simulink model "model2"  (R2021a)
settings: Solver=ode23s  StartTime=0.0  StopTime=0.1  MaxStep=1e-4  RelTol=1e-3
undefined symbols (not defined in the file): D1, Delta, lagging, pulse
libraries: spsVoltageMeasurementLib x23, spsThreePhaseTransformerTwoWindingsLib x22, spsUniversalBridgeLib x18, spsSeriesRLCBranchLib x15, spsRMSLib x13, spsCurrentMeasurementLib x12, spsThreePhaseProgrammableVoltageSourceLib x7, spsGroundLib x5, spsPulseGeneratorThyristor6PulseLib x5, simulink x5, spsThreePhaseTransformerThreeWindingsLib x4, spsControlledCurrentSourceLib x1
settings Model: Creator=Tasneem  LastModifiedBy=Tasneem

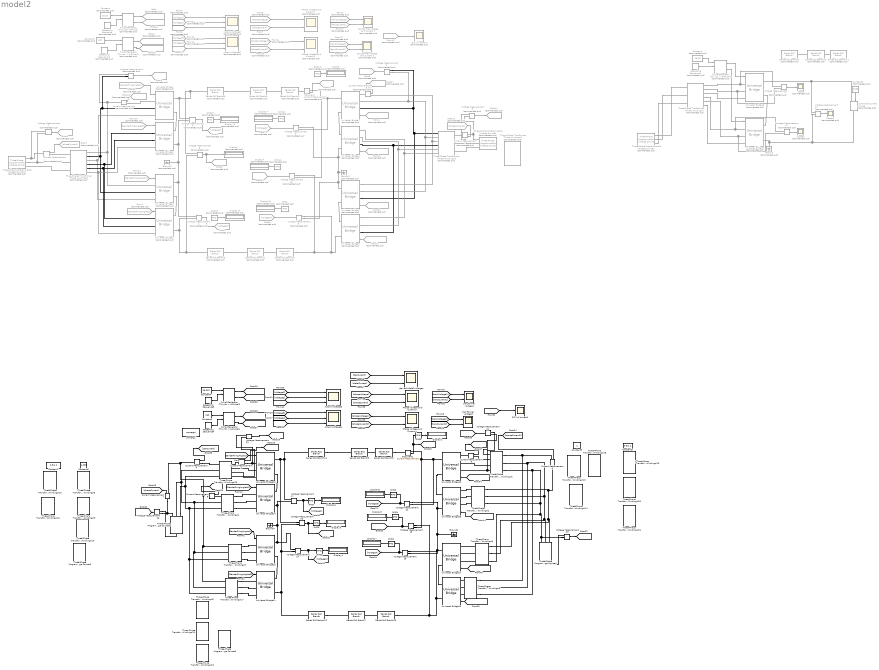
== system model2 ==
  Constant : Constant  Commented=on  Value=18.25
  Constant1 : Constant  Commented=on  Value=18.25
  Constant2 : Constant  Commented=on  Value=160
  Constant3 : Constant  Commented=on  Value=2835
  Constant4 : Constant  Value=28.357
  Constant5 : Constant  Value=160
  Constant6 : Constant  Value=1.025
  Constant7 : Constant  Value=0.9/1.1
  Constant8 : Constant
  Constant9 : Constant  Value=0.9/1.1
  Controlled Current Source : spsControlledCurrentSourceLib/Controlled Current Source  Commented=on  Initialize=on  Source_Type=AC  Amplitude=0  Phase=0  Frequency=0  Measurements=None
  Current Measurement{,1,3,10} (4 alike) : spsCurrentMeasurementLib/Current Measurement  Commented=on  PhasorSimulation=off  OutputType=Complex  PSBequivalent=0
  Current Measurement{2,4..8} (6 alike) : spsCurrentMeasurementLib/Current Measurement  PhasorSimulation=off  OutputType=Complex  PSBequivalent=0
  DC link current : Scope  Commented=on
  DC link current1 : Scope
  DCcurrent : spsCurrentMeasurementLib/Current Measurement  Commented=on  PhasorSimulation=off  OutputType=Complex  PSBequivalent=0
  DCcurrent1 : spsCurrentMeasurementLib/Current Measurement  PhasorSimulation=off  OutputType=Complex  PSBequivalent=0
  Display{,1,5,14..17} (7 alike) : Display  Commented=on
  Display{2..4,6..9} (7 alike) : Display
  From1 : From  Commented=on  GotoTag=SenderFiringAnglesD
  From10 : From  Commented=on  GotoTag=Voltage3
  From11 : From  Commented=on  GotoTag=VoltageSum2
  From12 : From  Commented=on  GotoTag=Voltage4
  From13 : From  Commented=on  GotoTag=transVoltage2
  From14 : From  Commented=on  GotoTag=phaseVoltage2
  From15 : From  Commented=on  GotoTag=phaseCurrent2
  From16 : From  Commented=on  GotoTag=DClinkCurrent
  From17 : From  Commented=on  GotoTag=transCurrent1
  From18 : From  Commented=on  GotoTag=transCurrent2
  From19 : From  Commented=on  GotoTag=ReceiverFiringAnglesD
  From2 : From  Commented=on  GotoTag=ReceiverFiringAnglesY
  From20 : From  Commented=on  GotoTag=ReceiverFiringAnglesY
  From22 : From  Commented=on  GotoTag=SenderFiringAnglesY
  From23 : From  Commented=on  GotoTag=SenderFiringAnglesY
  From24 : From  Commented=on  GotoTag=SenderFiringAnglesD
  From3 : From  Commented=on  GotoTag=ReceiverFiringAnglesD
  From4 : From  Commented=on  GotoTag=Voltage1
  From5 : From  Commented=on  GotoTag=transVoltage1
  From6 : From  Commented=on  GotoTag=phaseVoltage
  From7 : From  Commented=on  GotoTag=phaseCurrent
  From8 : From  Commented=on  GotoTag=VoltageSum1
  From9 : From  Commented=on  GotoTag=Voltage2
  Goto : Goto  Commented=on  GotoTag=SenderFiringAnglesY
  Goto1 : Goto  Commented=on  GotoTag=Voltage2
  Goto10 : Goto  Commented=on  GotoTag=Voltage3
  Goto11 : Goto  Commented=on  GotoTag=phaseVoltage2
  Goto12 : Goto  Commented=on  GotoTag=VoltageSum2
  Goto13 : Goto  Commented=on  GotoTag=phaseCurrent2
  Goto14 : Goto  Commented=on  GotoTag=DClinkCurrent
  Goto15 : Goto  Commented=on  GotoTag=transCurrent1
  Goto16 : Goto  Commented=on  GotoTag=SenderFiringAnglesD
  Goto17 : Goto  Commented=on  GotoTag=transCurrent2
  Goto18 : Goto  Commented=on  GotoTag=ReceiverFiringAnglesD
  Goto2 : Goto  Commented=on  GotoTag=ReceiverFiringAnglesY
  Goto3 : Goto  Commented=on  GotoTag=transVoltage1
  Goto4 : Goto  Commented=on  GotoTag=Voltage1
  Goto5 : Goto  Commented=on  GotoTag=phaseVoltage
  Goto6 : Goto  Commented=on  GotoTag=VoltageSum1
  Goto7 : Goto  Commented=on  GotoTag=phaseCurrent
  Goto8 : Goto  Commented=on  GotoTag=Voltage4
  Goto9 : Goto  Commented=on  GotoTag=transVoltage2
  Ground : spsGroundLib/Ground  Commented=on  LConnTagsString=a
  Ground1 : spsGroundLib/Ground  Commented=on  LConnTagsString=a
  Ground2 : spsGroundLib/Ground  LConnTagsString=a
  Ground3 : spsGroundLib/Ground  Commented=on  LConnTagsString=a
  Ground4 : spsGroundLib/Ground  LConnTagsString=a
  Phase Voltage and Current 1 : Scope  Commented=on  NumInputPorts=2
  Phase Voltage and Current 2 : Scope  Commented=on  NumInputPorts=2
  Phase Voltage and Current 3 : Scope  NumInputPorts=2
  Phase Voltage and Current 4 : Scope  NumInputPorts=2
  "Pulse Generator (Thyristor, 6-Pulse)" : spsPulseGeneratorThyristor6PulseLib/Pulse Generator (Thyristor, 6-Pulse)  Commented=on  GenType=12-pulse  Delta=D1 (lagging)  pwidth=60  Double_Pulse=on  Ts=0
      settings: SourceProductBaseCode=PS
  "Pulse Generator (Thyristor, 6-Pulse)1" : spsPulseGeneratorThyristor6PulseLib/Pulse Generator (Thyristor, 6-Pulse)  Commented=on  GenType=12-pulse  Delta=D1 (lagging)  pwidth=60  Double_Pulse=on  Ts=0
      settings: SourceProductBaseCode=PS
  "Pulse Generator (Thyristor, 6-Pulse)2" : spsPulseGeneratorThyristor6PulseLib/Pulse Generator (Thyristor, 6-Pulse)  Commented=on  GenType=12-pulse  Delta=D1 (lagging)  pwidth=60  Double_Pulse=on  Ts=0
      settings: SourceProductBaseCode=PS
  "Pulse Generator (Thyristor, 6-Pulse)3" : spsPulseGeneratorThyristor6PulseLib/Pulse Generator (Thyristor, 6-Pulse)  GenType=12-pulse  Delta=D1 (lagging)  pwidth=60  Double_Pulse=on  Ts=0
      settings: SourceProductBaseCode=PS
  "Pulse Generator (Thyristor, 6-Pulse)4" : spsPulseGeneratorThyristor6PulseLib/Pulse Generator (Thyristor, 6-Pulse)  GenType=12-pulse  Delta=D1 (lagging)  pwidth=60  Double_Pulse=on  Ts=0
      settings: SourceProductBaseCode=PS
  RMS1 : spsRMSLib/RMS  Commented=on  TrueRMS=on  Freq=60  RMSInit=120  Ts=0
  RMS10 : spsRMSLib/RMS  Commented=on  TrueRMS=on  Freq=50  RMSInit=120  Ts=0
  RMS11 : spsRMSLib/RMS  Commented=on  TrueRMS=on  Freq=60  RMSInit=120  Ts=0
  RMS12 : spsRMSLib/RMS  Commented=on  TrueRMS=on  Freq=60  RMSInit=120  Ts=0
  RMS13 : spsRMSLib/RMS  Commented=on  TrueRMS=on  Freq=50  RMSInit=120  Ts=0
  RMS15 : spsRMSLib/RMS  Commented=on  TrueRMS=on  Freq=50  RMSInit=120  Ts=0
  RMS2 : spsRMSLib/RMS  TrueRMS=on  Freq=60  RMSInit=120  Ts=0
  RMS{3,6..7,9} (4 alike) : spsRMSLib/RMS  TrueRMS=on  Freq=50  RMSInit=120  Ts=0
  RMS4 : spsRMSLib/RMS  TrueRMS=on  Freq=60  RMSInit=120  Ts=0
  RMS5 : spsRMSLib/RMS  TrueRMS=on  Freq=60  RMSInit=120  Ts=0
  Repeating Sequence : simulink/Sources/Repeating Sequence  Commented=on  rep_seq_t=[0 1/50]  rep_seq_y=[0 2*pi]
  Repeating Sequence1 : simulink/Sources/Repeating Sequence  Commented=on  rep_seq_t=[0 1/50]  rep_seq_y=[0 2*pi]
  Repeating Sequence2 : simulink/Sources/Repeating Sequence  Commented=on  rep_seq_t=[0 1/60]  rep_seq_y=[0 2*pi]
  Repeating Sequence3 : simulink/Sources/Repeating Sequence  rep_seq_t=[0 1/50]  rep_seq_y=[0 2*pi]
  Repeating Sequence4 : simulink/Sources/Repeating Sequence  rep_seq_t=[0 1/60]  rep_seq_y=[0 2*pi]
  Scope : Scope  Commented=on
  Scope1 : Scope  Commented=on
  Scope2 : Scope  Commented=on
  Series RLC Branch : spsSeriesRLCBranchLib/Series RLC Branch  Commented=on  LConnTagsString=__new0  RConnTagsString=__new0  BranchType=R  Resistance=10  Inductance=1e-3  SetiL0=off  InitialCurrent=0  Capacitance=1e-6  Setx0=off  InitialVoltage=0  Measurements=None
  Series RLC Branch1 : spsSeriesRLCBranchLib/Series RLC Branch  Commented=on  LConnTagsString=__new0  RConnTagsString=__new0  BranchType=R  Resistance=10  Inductance=1e-3  SetiL0=off  InitialCurrent=0  Capacitance=1e-6  Setx0=off  InitialVoltage=0  Measurements=None
  Series RLC Branch10 : spsSeriesRLCBranchLib/Series RLC Branch  Commented=on  LConnTagsString=__new0  RConnTagsString=__new0  BranchType=R  Resistance=10  Inductance=1e-3  SetiL0=off  InitialCurrent=0  Capacitance=1e-6  Setx0=off  InitialVoltage=0  Measurements=None
  Series RLC Branch11 : spsSeriesRLCBranchLib/Series RLC Branch  Commented=on  LConnTagsString=__new0  RConnTagsString=__new0  BranchType=L  Resistance=1  Inductance=0.1  SetiL0=off  InitialCurrent=0  Capacitance=1e-6  Setx0=off  InitialVoltage=0  Measurements=None
  Series RLC Branch{8,12..14} (4 alike) : spsSeriesRLCBranchLib/Series RLC Branch  LConnTagsString=__new0  RConnTagsString=__new0  BranchType=L  Resistance=10  Inductance=0.1  SetiL0=off  InitialCurrent=0  Capacitance=1e-6  Setx0=off  InitialVoltage=0  Measurements=None
  Series RLC Branch{2,4..6} (4 alike) : spsSeriesRLCBranchLib/Series RLC Branch  Commented=on  LConnTagsString=__new0  RConnTagsString=__new0  BranchType=L  Resistance=10  Inductance=0.1  SetiL0=off  InitialCurrent=0  Capacitance=1e-6  Setx0=off  InitialVoltage=0  Measurements=None
  Series RLC Branch3 : spsSeriesRLCBranchLib/Series RLC Branch  LConnTagsString=__new0  RConnTagsString=__new0  BranchType=R  Resistance=10  Inductance=1e-3  SetiL0=off  InitialCurrent=0  Capacitance=1e-6  Setx0=off  InitialVoltage=0  Measurements=None
  Series RLC Branch7 : spsSeriesRLCBranchLib/Series RLC Branch  LConnTagsString=__new0  RConnTagsString=__new0  BranchType=R  Resistance=10  Inductance=1e-3  SetiL0=off  InitialCurrent=0  Capacitance=1e-6  Setx0=off  InitialVoltage=0  Measurements=None
  Series RLC Branch9 : spsSeriesRLCBranchLib/Series RLC Branch  Commented=on  LConnTagsString=__new0  RConnTagsString=__new0  BranchType=L  Resistance=1  Inductance=0.1  SetiL0=off  InitialCurrent=0  Capacitance=1e-6  Setx0=off  InitialVoltage=0  Measurements=None
  Three-Phase Programmable Voltage Source1 : spsThreePhaseProgrammableVoltageSourceLib/Three-Phase Programmable Voltage Source  Commented=on  PositiveSequence="[22e3*1.025  0 50]"  VariationEntity=None  VariationType=Table of time-amplitude pairs  VariationTypeAlt=Step  VariationStep=0.5  VariationRate=10  VariationMagnitude=0.3  VariationFrequency=2  VariationTiming=[1 2]  VariationPhaseA=off  Amplitudes=[1 0.8 1.2 1.0]  TimeValues=[0 0.1 0.15 0.2]  HarmonicGeneration=off  HarmonicA=[3 0.2 -25 0]  HarmonicB=[2 0.15 35 2]  Timing="[0.05  3]"  BusType=swing  Pref=0  Qref=0  Qmin=-inf  Qmax=inf
  Three-Phase Programmable Voltage Source10 : spsThreePhaseProgrammableVoltageSourceLib/Three-Phase Programmable Voltage Source  Commented=on  PositiveSequence="[22e3*1.025  0 50]"  VariationEntity=None  VariationType=Table of time-amplitude pairs  VariationTypeAlt=Step  VariationStep=0.5  VariationRate=10  VariationMagnitude=0.3  VariationFrequency=2  VariationTiming=[1 2]  VariationPhaseA=off  Amplitudes=[1 0.8 1.2 1.0]  TimeValues=[0 0.1 0.15 0.2]  HarmonicGeneration=off  HarmonicA=[3 0.2 -25 0]  HarmonicB=[2 0.15 35 2]  Timing="[0.05  3]"  BusType=swing  Pref=0  Qref=0  Qmin=-inf  Qmax=inf
  Three-Phase Programmable Voltage Source2 : spsThreePhaseProgrammableVoltageSourceLib/Three-Phase Programmable Voltage Source  PositiveSequence="[22e3  0 50]"  VariationEntity=None  VariationType=Table of time-amplitude pairs  VariationTypeAlt=Step  VariationStep=0.5  VariationRate=10  VariationMagnitude=0.3  VariationFrequency=2  VariationTiming=[1 2]  VariationPhaseA=off  Amplitudes=[1 0.8 1.2 1.0]  TimeValues=[0 0.1 0.15 0.2]  HarmonicGeneration=off  HarmonicA=[3 0.2 -25 0]  HarmonicB=[2 0.15 35 2]  Timing="[0.05  3]"  BusType=swing  Pref=0  Qref=0  Qmin=-inf  Qmax=inf
  Three-Phase Programmable Voltage Source3 : spsThreePhaseProgrammableVoltageSourceLib/Three-Phase Programmable Voltage Source  Commented=on  PositiveSequence="[20e3  0 60]"  VariationEntity=None  VariationType=Table of time-amplitude pairs  VariationTypeAlt=Step  VariationStep=0.5  VariationRate=10  VariationMagnitude=0.3  VariationFrequency=2  VariationTiming=[1 2]  VariationPhaseA=off  Amplitudes=[1 0.8 1.2 1.0]  TimeValues=[0 0.1 0.15 0.2]  HarmonicGeneration=off  HarmonicA=[3 0.2 -25 0]  HarmonicB=[2 0.15 35 2]  Timing="[0.05  3]"  BusType=swing  Pref=0  Qref=0  Qmin=-inf  Qmax=inf
  Three-Phase Programmable Voltage Source4 : spsThreePhaseProgrammableVoltageSourceLib/Three-Phase Programmable Voltage Source  PositiveSequence="[20e3  0 60]"  VariationEntity=None  VariationType=Table of time-amplitude pairs  VariationTypeAlt=Step  VariationStep=0.5  VariationRate=10  VariationMagnitude=0.3  VariationFrequency=2  VariationTiming=[1 2]  VariationPhaseA=off  Amplitudes=[1 0.8 1.2 1.0]  TimeValues=[0 0.1 0.15 0.2]  HarmonicGeneration=off  HarmonicA=[3 0.2 -25 0]  HarmonicB=[2 0.15 35 2]  Timing="[0.05  3]"  BusType=swing  Pref=0  Qref=0  Qmin=-inf  Qmax=inf
  Three-Phase Programmable Voltage Source5 : spsThreePhaseProgrammableVoltageSourceLib/Three-Phase Programmable Voltage Source  PositiveSequence="[22e3*1.025  0 50]"  VariationEntity=None  VariationType=Table of time-amplitude pairs  VariationTypeAlt=Step  VariationStep=0.5  VariationRate=10  VariationMagnitude=0.3  VariationFrequency=2  VariationTiming=[1 2]  VariationPhaseA=off  Amplitudes=[1 0.8 1.2 1.0]  TimeValues=[0 0.1 0.15 0.2]  HarmonicGeneration=off  HarmonicA=[3 0.2 -25 0]  HarmonicB=[2 0.15 35 2]  Timing="[0.05  3]"  BusType=swing  Pref=0  Qref=0  Qmin=-inf  Qmax=inf
  Three-Phase Programmable Voltage Source6 : spsThreePhaseProgrammableVoltageSourceLib/Three-Phase Programmable Voltage Source  PositiveSequence="[22e3  0 50]"  VariationEntity=None  VariationType=Table of time-amplitude pairs  VariationTypeAlt=Step  VariationStep=0.5  VariationRate=10  VariationMagnitude=0.3  VariationFrequency=2  VariationTiming=[1 2]  VariationPhaseA=off  Amplitudes=[1 0.8 1.2 1.0]  TimeValues=[0 0.1 0.15 0.2]  HarmonicGeneration=off  HarmonicA=[3 0.2 -25 0]  HarmonicB=[2 0.15 35 2]  Timing="[0.05  3]"  BusType=swing  Pref=0  Qref=0  Qmin=-inf  Qmax=inf
  Three-Phase Transformer (Three Windings)1 : spsThreePhaseTransformerThreeWindingsLib/Three-Phase Transformer (Three Windings)  Commented=on  Winding1Connection=Y  Winding2Connection=Y  Winding3Connection=Delta (D1)  CoreType=Three single-phase transformers  SetSaturation=off  Hysteresis=off  DataFile='hysteresis'  SetInitialFlux=off  Measurements=None  UNITS=SI  NominalPower=[ 1600e6 , 50 ]  Winding1=[22e3 0 0]  Winding2=[220e3 0 0]  Winding3=[220e3*sqrt(3) 0.001 0]  Rm=inf  Lm=inf  L0=0.5  Saturation=[0 0;4.2658 1910.3;1777.4 2419.7]  InitialFluxes=[0 87.9108143390969 87.9108143390969]  BreakLoop=off  DiscreteSolver=Trapezoidal iterative  DataType=on  TransfoNumber=1
      settings: SourceProductBaseCode=PS
  Three-Phase Transformer (Three Windings)2 : spsThreePhaseTransformerThreeWindingsLib/Three-Phase Transformer (Three Windings)  Commented=on  Winding1Connection=Y  Winding2Connection=Y  Winding3Connection=Delta (D1)  CoreType=Three single-phase transformers  SetSaturation=off  Hysteresis=off  DataFile='hysteresis'  SetInitialFlux=off  Measurements=None  UNITS=SI  NominalPower=[ 1600e6 , 50 ]  Winding1=[22e3 0 0]  Winding2=[220e3 0 0]  Winding3=[220e3*sqrt(3) 0.001 0]  Rm=inf  Lm=inf  L0=0.5  Saturation=[0 0;4.2658 1910.3;1777.4 2419.7]  InitialFluxes=[0 87.9108143390969 87.9108143390969]  BreakLoop=off  DiscreteSolver=Trapezoidal iterative  DataType=on  TransfoNumber=1
      settings: SourceProductBaseCode=PS
  Three-Phase Transformer (Three Windings)3 : spsThreePhaseTransformerThreeWindingsLib/Three-Phase Transformer (Three Windings)  Commented=on  Winding1Connection=Y  Winding2Connection=Y  Winding3Connection=Delta (D1)  CoreType=Three single-phase transformers  SetSaturation=off  Hysteresis=off  DataFile='hysteresis'  SetInitialFlux=off  Measurements=None  UNITS=SI  NominalPower=[ 18000e6 , 60 ]  Winding1=[20e3 0 0]  Winding2=[200e3 0 0]  Winding3=[200e3*sqrt(3) 0.0001 0]  Rm=inf  Lm=inf  L0=0.5  Saturation=[0 0;0.66653 1910.3;277.72 2419.7]  InitialFluxes=[-43.3164889574264 21.6582444787132 21.6582444787132]  BreakLoop=off  DiscreteSolver=Trapezoidal iterative  DataType=on  TransfoNumber=1
      settings: SourceProductBaseCode=PS
  Three-Phase Transformer (Three Windings)4 : spsThreePhaseTransformerThreeWindingsLib/Three-Phase Transformer (Three Windings)  Commented=on  Winding1Connection=Y  Winding2Connection=Y  Winding3Connection=Delta (D1)  CoreType=Three single-phase transformers  SetSaturation=off  Hysteresis=off  DataFile='hysteresis'  SetInitialFlux=off  Measurements=None  UNITS=SI  NominalPower=[ 1600e6 , 60 ]  Winding1=[20e3 0 0]  Winding2=[200e3 0 0]  Winding3=[200e3*sqrt(3) 0.001 0]  Rm=inf  Lm=inf  L0=0.5  Saturation=[0 0;4.2658 1910.3;1777.4 2419.7]  InitialFluxes=[0 64.9747334361397 64.9747334361397]  BreakLoop=off  DiscreteSolver=Trapezoidal iterative  DataType=on  TransfoNumber=1
      settings: SourceProductBaseCode=PS
  Three-Phase Transformer (Two Windings)1 : spsThreePhaseTransformerTwoWindingsLib/Three-Phase Transformer (Two Windings)  Winding1Connection=Yn  Winding2Connection=Y  CoreType=Three single-phase transformers  SetSaturation=off  Hysteresis=off  DataFile='hysteresis'  SetInitialFlux=off  Measurements=None  UNITS=SI  NominalPower=[ 800e6 , 60 ]  Winding1=[200e3 0.001 0]  Winding2=[20e3 0.001 0]  Rm=inf  Lm=inf  L0=0.5  Saturation=[0 0;17.636 519.8;7348.5 658.41]  InitialFluxes=[0 714.722067624574 714.722315656474]  BreakLoop=off  DiscreteSolver=Trapezoidal iterative  DataType=on  TransfoNumber=1
  Three-Phase Transformer (Two Windings)10 : spsThreePhaseTransformerTwoWindingsLib/Three-Phase Transformer (Two Windings)  Winding1Connection=Y  Winding2Connection=Y  CoreType=Three single-phase transformers  SetSaturation=off  Hysteresis=off  DataFile='hysteresis'  SetInitialFlux=off  Measurements=None  UNITS=SI  NominalPower=[ 800e6 , 50 ]  Winding1=[22e3*1.025 1e-6 0]  Winding2=[220e3*1.025 1e-6 0]  Rm=inf  Lm=inf  L0=0.00044961  Saturation=[0 0;156.42 70.329;65175 89.083]  InitialFluxes=[0 85.766648119398 85.766648119398]  BreakLoop=off  DiscreteSolver=Trapezoidal iterative  DataType=on  TransfoNumber=1
  Three-Phase Transformer (Two Windings)11 : spsThreePhaseTransformerTwoWindingsLib/Three-Phase Transformer (Two Windings)  Winding1Connection=Y  Winding2Connection=Delta (D1)  CoreType=Three single-phase transformers  SetSaturation=off  Hysteresis=off  DataFile='hysteresis'  SetInitialFlux=off  Measurements=None  UNITS=SI  NominalPower=[ 800e6 , 50 ]  Winding1=[22e3 1e-6 0]  Winding2=[220e3 1e-6 0]  Rm=inf  Lm=inf  L0=0.00044961  Saturation=[0 0;156.42 70.329;65175 89.083]  InitialFluxes=[0 85.766648119398 85.766648119398]  BreakLoop=off  DiscreteSolver=Trapezoidal iterative  DataType=on  TransfoNumber=1
  Three-Phase Transformer (Two Windings)12 : spsThreePhaseTransformerTwoWindingsLib/Three-Phase Transformer (Two Windings)  Winding1Connection=Y  Winding2Connection=Y  CoreType=Three single-phase transformers  SetSaturation=off  Hysteresis=off  DataFile='hysteresis'  SetInitialFlux=off  Measurements=None  UNITS=SI  NominalPower=[ 800e6 , 50 ]  Winding1=[22e3 1e-6 0]  Winding2=[220e3 1e-6 0]  Rm=inf  Lm=inf  L0=0.00044961  Saturation=[0 0;156.42 70.329;65175 89.083]  InitialFluxes=[0 85.766648119398 85.766648119398]  BreakLoop=off  DiscreteSolver=Trapezoidal iterative  DataType=on  TransfoNumber=1
  Three-Phase Transformer (Two Windings)13 : spsThreePhaseTransformerTwoWindingsLib/Three-Phase Transformer (Two Windings)  Winding1Connection=Y  Winding2Connection=Y  CoreType=Three single-phase transformers  SetSaturation=off  Hysteresis=off  DataFile='hysteresis'  SetInitialFlux=off  Measurements=None  UNITS=SI  NominalPower=[ 800e6 , 60 ]  Winding1=[200e3 1e-6 0]  Winding2=[20e3 1e-6 0]  Rm=inf  Lm=inf  L0=0.5  Saturation=[0 0;17.636 519.8;7348.5 658.41]  InitialFluxes=[0 714.722067624574 714.722315656474]  BreakLoop=off  DiscreteSolver=Trapezoidal iterative  DataType=on  TransfoNumber=1
  Three-Phase Transformer (Two Windings)14 : spsThreePhaseTransformerTwoWindingsLib/Three-Phase Transformer (Two Windings)  Winding1Connection=Delta (D1)  Winding2Connection=Y  CoreType=Three single-phase transformers  SetSaturation=off  Hysteresis=off  DataFile='hysteresis'  SetInitialFlux=off  Measurements=None  UNITS=SI  NominalPower=[ 800e6 , 60 ]  Winding1=[200e3 1e-6 0]  Winding2=[20e3 1e-6 0]  Rm=inf  Lm=inf  L0=0.5  Saturation=[0 0;17.636 519.8;7348.5 658.41]  InitialFluxes=[0 714.722067624574 714.722315656474]  BreakLoop=off  DiscreteSolver=Trapezoidal iterative  DataType=on  TransfoNumber=1
  Three-Phase Transformer (Two Windings)15 : spsThreePhaseTransformerTwoWindingsLib/Three-Phase Transformer (Two Windings)  Winding1Connection=Y  Winding2Connection=Yn  CoreType=Three single-phase transformers  SetSaturation=off  Hysteresis=off  DataFile='hysteresis'  SetInitialFlux=off  Measurements=None  UNITS=SI  NominalPower=[ 800e6 , 50 ]  Winding1=[22e3 1e-6 0]  Winding2=[220e3*0.9 1e-6 0]  Rm=inf  Lm=inf  L0=0.00044961  Saturation=[0 0;156.42 70.329;65175 89.083]  InitialFluxes=[0 85.766648119398 85.766648119398]  BreakLoop=off  DiscreteSolver=Trapezoidal iterative  DataType=on  TransfoNumber=1
  Three-Phase Transformer (Two Windings)16 : spsThreePhaseTransformerTwoWindingsLib/Three-Phase Transformer (Two Windings)  Winding1Connection=Y  Winding2Connection=Delta (D1)  CoreType=Three single-phase transformers  SetSaturation=off  Hysteresis=off  DataFile='hysteresis'  SetInitialFlux=off  Measurements=None  UNITS=SI  NominalPower=[ 800e6 , 50 ]  Winding1=[22e3 1e-6 0]  Winding2=[220e3*0.9 1e-6 0]  Rm=inf  Lm=inf  L0=0.00044961  Saturation=[0 0;156.42 70.329;65175 89.083]  InitialFluxes=[0 85.766648119398 85.766648119398]  BreakLoop=off  DiscreteSolver=Trapezoidal iterative  DataType=on  TransfoNumber=1
  Three-Phase Transformer (Two Windings)17 : spsThreePhaseTransformerTwoWindingsLib/Three-Phase Transformer (Two Windings)  Winding1Connection=Y  Winding2Connection=Delta (D1)  CoreType=Three single-phase transformers  SetSaturation=off  Hysteresis=off  DataFile='hysteresis'  SetInitialFlux=off  Measurements=None  UNITS=SI  NominalPower=[ 800e6 , 50 ]  Winding1=[22e3 1e-6 0]  Winding2=[220e3 1e-6 0]  Rm=inf  Lm=inf  L0=0.00044961  Saturation=[0 0;156.42 70.329;65175 89.083]  InitialFluxes=[0 85.766648119398 85.766648119398]  BreakLoop=off  DiscreteSolver=Trapezoidal iterative  DataType=on  TransfoNumber=1
  Three-Phase Transformer (Two Windings)18 : spsThreePhaseTransformerTwoWindingsLib/Three-Phase Transformer (Two Windings)  Winding1Connection=Yn  Winding2Connection=Y  CoreType=Three single-phase transformers  SetSaturation=off  Hysteresis=off  DataFile='hysteresis'  SetInitialFlux=off  Measurements=None  UNITS=SI  NominalPower=[ 800e6 , 60 ]  Winding1=[200e3 1e-6 0]  Winding2=[20e3 1e-6 0]  Rm=inf  Lm=inf  L0=0.5  Saturation=[0 0;17.636 519.8;7348.5 658.41]  InitialFluxes=[0 714.722067624574 714.722315656474]  BreakLoop=off  DiscreteSolver=Trapezoidal iterative  DataType=on  TransfoNumber=1
  Three-Phase Transformer (Two Windings)19 : spsThreePhaseTransformerTwoWindingsLib/Three-Phase Transformer (Two Windings)  Winding1Connection=Yn  Winding2Connection=Y  CoreType=Three single-phase transformers  SetSaturation=off  Hysteresis=off  DataFile='hysteresis'  SetInitialFlux=off  Measurements=None  UNITS=SI  NominalPower=[ 800e6 , 60 ]  Winding1=[200e3*1.1 1e-6 0]  Winding2=[20e3 1e-6 0]  Rm=inf  Lm=inf  L0=0.5  Saturation=[0 0;17.636 519.8;7348.5 658.41]  InitialFluxes=[0 714.722067624574 714.722315656474]  BreakLoop=off  DiscreteSolver=Trapezoidal iterative  DataType=on  TransfoNumber=1
  Three-Phase Transformer (Two Windings)2 : spsThreePhaseTransformerTwoWindingsLib/Three-Phase Transformer (Two Windings)  Winding1Connection=Delta (D1)  Winding2Connection=Y  CoreType=Three single-phase transformers  SetSaturation=off  Hysteresis=off  DataFile='hysteresis'  SetInitialFlux=off  Measurements=None  UNITS=SI  NominalPower=[ 800e6 , 60 ]  Winding1=[200e3 1e-6 0]  Winding2=[20e3 1e-6 0]  Rm=inf  Lm=inf  L0=0.5  Saturation=[0 0;17.636 519.8;7348.5 658.41]  InitialFluxes=[0 714.722067624574 714.722315656474]  BreakLoop=off  DiscreteSolver=Trapezoidal iterative  DataType=on  TransfoNumber=1
  Three-Phase Transformer (Two Windings)20 : spsThreePhaseTransformerTwoWindingsLib/Three-Phase Transformer (Two Windings)  Winding1Connection=Delta (D1)  Winding2Connection=Y  CoreType=Three single-phase transformers  SetSaturation=off  Hysteresis=off  DataFile='hysteresis'  SetInitialFlux=off  Measurements=None  UNITS=SI  NominalPower=[ 800e6 , 60 ]  Winding1=[200e3*1.1 1e-6 0]  Winding2=[20e3 1e-6 0]  Rm=inf  Lm=inf  L0=0.5  Saturation=[0 0;17.636 519.8;7348.5 658.41]  InitialFluxes=[0 714.722067624574 714.722315656474]  BreakLoop=off  DiscreteSolver=Trapezoidal iterative  DataType=on  TransfoNumber=1
  Three-Phase Transformer (Two Windings)21 : spsThreePhaseTransformerTwoWindingsLib/Three-Phase Transformer (Two Windings)  Winding1Connection=Y  Winding2Connection=Y  CoreType=Three single-phase transformers  SetSaturation=off  Hysteresis=off  DataFile='hysteresis'  SetInitialFlux=off  Measurements=None  UNITS=SI  NominalPower=[ 800e6 , 60 ]  Winding1=[200e3*1.1 0.0001 0]  Winding2=[20e3 0.0001 0]  Rm=inf  Lm=inf  L0=0.5  Saturation=[0 0;17.636 519.8;7348.5 658.41]  InitialFluxes=[0 714.722067624574 714.722315656474]  BreakLoop=off  DiscreteSolver=Trapezoidal iterative  DataType=on  TransfoNumber=1
  Three-Phase Transformer (Two Windings)23 : spsThreePhaseTransformerTwoWindingsLib/Three-Phase Transformer (Two Windings)  Winding1Connection=Y  Winding2Connection=Yn  CoreType=Three single-phase transformers  SetSaturation=off  Hysteresis=off  DataFile='hysteresis'  SetInitialFlux=off  Measurements=None  UNITS=SI  NominalPower=[ 800e6 , 50 ]  Winding1=[22e3 1e-6 0]  Winding2=[220e3 1e-6 0]  Rm=inf  Lm=inf  L0=0.00044961  Saturation=[0 0;156.42 70.329;65175 89.083]  InitialFluxes=[0 85.766648119398 85.766648119398]  BreakLoop=off  DiscreteSolver=Trapezoidal iterative  DataType=on  TransfoNumber=1
  Three-Phase Transformer (Two Windings)3 : spsThreePhaseTransformerTwoWindingsLib/Three-Phase Transformer (Two Windings)  Winding1Connection=Y  Winding2Connection=Yn  CoreType=Three single-phase transformers  SetSaturation=off  Hysteresis=off  DataFile='hysteresis'  SetInitialFlux=off  Measurements=None  UNITS=SI  NominalPower=[ 800e6 , 50 ]  Winding1=[22e3 1e-6 0]  Winding2=[220e3 1e-6 0]  Rm=inf  Lm=inf  L0=0.00044961  Saturation=[0 0;156.42 70.329;65175 89.083]  InitialFluxes=[0 85.766648119398 85.766648119398]  BreakLoop=off  DiscreteSolver=Trapezoidal iterative  DataType=on  TransfoNumber=1
  Three-Phase Transformer (Two Windings)4 : spsThreePhaseTransformerTwoWindingsLib/Three-Phase Transformer (Two Windings)  Winding1Connection=Y  Winding2Connection=Delta (D1)  CoreType=Three single-phase transformers  SetSaturation=off  Hysteresis=off  DataFile='hysteresis'  SetInitialFlux=off  Measurements=None  UNITS=SI  NominalPower=[ 800e6 , 50 ]  Winding1=[22e3 1e-6 0]  Winding2=[220e3 1e-6 0]  Rm=inf  Lm=inf  L0=0.00044961  Saturation=[0 0;156.42 70.329;65175 89.083]  InitialFluxes=[0 85.766648119398 85.766648119398]  BreakLoop=off  DiscreteSolver=Trapezoidal iterative  DataType=on  TransfoNumber=1
  Three-Phase Transformer (Two Windings)5 : spsThreePhaseTransformerTwoWindingsLib/Three-Phase Transformer (Two Windings)  Winding1Connection=Y  Winding2Connection=Yn  CoreType=Three single-phase transformers  SetSaturation=off  Hysteresis=off  DataFile='hysteresis'  SetInitialFlux=off  Measurements=None  UNITS=SI  NominalPower=[ 800e6 , 50 ]  Winding1=[22e3*1.025 1e-6 0]  Winding2=[220e3*1.025 1e-6 0]  Rm=inf  Lm=inf  L0=0.00044961  Saturation=[0 0;156.42 70.329;65175 89.083]  InitialFluxes=[0 85.766648119398 85.766648119398]  BreakLoop=off  DiscreteSolver=Trapezoidal iterative  DataType=on  TransfoNumber=1
  Three-Phase Transformer (Two Windings)6 : spsThreePhaseTransformerTwoWindingsLib/Three-Phase Transformer (Two Windings)  Winding1Connection=Y  Winding2Connection=Y  CoreType=Three single-phase transformers  SetSaturation=off  Hysteresis=off  DataFile='hysteresis'  SetInitialFlux=off  Measurements=None  UNITS=SI  NominalPower=[ 800e6 , 60 ]  Winding1=[200e3 0.001 0]  Winding2=[20e3 0.001 0]  Rm=inf  Lm=inf  L0=0.5  Saturation=[0 0;17.636 519.8;7348.5 658.41]  InitialFluxes=[0 714.722067624574 714.722315656474]  BreakLoop=off  DiscreteSolver=Trapezoidal iterative  DataType=on  TransfoNumber=1
  Three-Phase Transformer (Two Windings)7 : spsThreePhaseTransformerTwoWindingsLib/Three-Phase Transformer (Two Windings)  Winding1Connection=Y  Winding2Connection=Y  CoreType=Three single-phase transformers  SetSaturation=off  Hysteresis=off  DataFile='hysteresis'  SetInitialFlux=off  Measurements=None  UNITS=SI  NominalPower=[ 800e6 , 50 ]  Winding1=[22e3 1e-6 0]  Winding2=[220e3 1e-6 0]  Rm=inf  Lm=inf  L0=0.00044961  Saturation=[0 0;156.42 70.329;65175 89.083]  InitialFluxes=[0 85.766648119398 85.766648119398]  BreakLoop=off  DiscreteSolver=Trapezoidal iterative  DataType=on  TransfoNumber=1
  Three-Phase Transformer (Two Windings)8 : spsThreePhaseTransformerTwoWindingsLib/Three-Phase Transformer (Two Windings)  Winding1Connection=Delta (D1)  Winding2Connection=Y  CoreType=Three single-phase transformers  SetSaturation=off  Hysteresis=off  DataFile='hysteresis'  SetInitialFlux=off  Measurements=None  UNITS=SI  NominalPower=[ 800e6 , 60 ]  Winding1=[200e3 1e-6 0]  Winding2=[20e3 1e-6 0]  Rm=inf  Lm=inf  L0=0.5  Saturation=[0 0;17.636 519.8;7348.5 658.41]  InitialFluxes=[0 714.722067624574 714.722315656474]  BreakLoop=off  DiscreteSolver=Trapezoidal iterative  DataType=on  TransfoNumber=1
  Three-Phase Transformer (Two Windings)9 : spsThreePhaseTransformerTwoWindingsLib/Three-Phase Transformer (Two Windings)  Winding1Connection=Y  Winding2Connection=Delta (D1)  CoreType=Three single-phase transformers  SetSaturation=off  Hysteresis=off  DataFile='hysteresis'  SetInitialFlux=off  Measurements=None  UNITS=SI  NominalPower=[ 800e6 , 50 ]  Winding1=[22e3*1.025 1e-6 0]  Winding2=[220e3*1.025 1e-6 0]  Rm=inf  Lm=inf  L0=0.00044961  Saturation=[0 0;156.42 70.329;65175 89.083]  InitialFluxes=[0 85.766648119398 85.766648119398]  BreakLoop=off  DiscreteSolver=Trapezoidal iterative  DataType=on  TransfoNumber=1
  Universal Bridge{,1..9} (10 alike) : spsUniversalBridgeLib/Universal Bridge  Commented=on  Arms=3  SnubberResistance=1e5  SnubberCapacitance=inf  Device=Thyristors  Ron=1e-9  Lon=0  ForwardVoltages="[  0  0  ]"  ForwardVoltage=0  GTOparameters=[ 10e-6 , 20e-6 ]  IGBTparameters=[ 1e-6 , 2e-6 ]  Measurements=None  Measurements_2=None  converterType=Rectifier
  Universal Bridge{10..17} (8 alike) : spsUniversalBridgeLib/Universal Bridge  Arms=3  SnubberResistance=1e5  SnubberCapacitance=inf  Device=Thyristors  Ron=1e-9  Lon=0  ForwardVoltages="[  0  0  ]"  ForwardVoltage=0  GTOparameters=[ 10e-6 , 20e-6 ]  IGBTparameters=[ 1e-6 , 2e-6 ]  Measurements=None  Measurements_2=None  converterType=Rectifier
  Voltage Measurement{,1..12} (13 alike) : spsVoltageMeasurementLib/Voltage Measurement  Commented=on  PhasorSimulation=off  OutputType=Complex  PSBequivalent=0
  Voltage Measurement{13..22} (10 alike) : spsVoltageMeasurementLib/Voltage Measurement  PhasorSimulation=off  OutputType=Complex  PSBequivalent=0
  output voltages1 : Scope  Commented=on  NumInputPorts=3
  output voltages2 : Scope  Commented=on  NumInputPorts=3
  output voltages3 : Scope  NumInputPorts=3
  output voltages4 : Scope  NumInputPorts=3
  powergui : spspowerguiLib/powergui  Priority=1  SimulationMode=Discrete  SampleTime=1e-6  frequency=60  Iterations=50  frequencyindice=0  Pbase=100e6  ErrMax=1e-4  UnitsV=kV  UnitsW=MW  buscounter=0  FunctionMessages=off  echomessages=off  EnableUseOfTLC=off  CurrentSourceSwitches=off  DisableSnubberDevices=off  DisableRonSwitches=off  DisableVfSwitches=off  DisplayEquations=off  AutomaticDiscreteSolvers=off  SolverType=Tustin/Backward Euler (TBE)  Interpol=off  ExternalGateDelay=off  methode=off  Ts=100  x0status=blocks  SPID=on  SwTol=0  HookPort=off  NonlinearTolerance=1e-4  nMaxIteration=100  ContinueOnMaxIteration=off  RestoreLinks=warning  ResistiveCurrentMeasurement=off  Frange=[0:2:500]  Ylog=off  Xlog=on  ShowGrid=off  save=off  variable=ZData  structure=0  ZoomFFT=off  StartTime=0.0  cycles=1  DisplayStyle=1  fundamental=60  FreqAxis=off  MaxFrequency=1000  frequencyindicesteady=1  RmsSteady=1  display=off
  star and delta voltages : Scope  NumInputPorts=2
  transformer voltage and current 1 : Scope  Commented=on  NumInputPorts=2
  transformer voltage and current 2 : Scope  Commented=on  NumInputPorts=2
  transformer voltage1 : Scope  NumInputPorts=2
  transformer voltage2 : Scope  NumInputPorts=2
  wires:
  Voltage Measurement2/1 -> Goto5/1
  RMS11/1 -> Display5/1
  RMS15/1 -> Display15/1
  RMS10/1 -> Display14/1
  Current Measurement10/1 -> Goto17/1
  RMS1/1 -> Display16/1
  From3/1 -> Universal Bridge3/1
  DCcurrent/1 -> Goto14/1
  From15/1 -> Phase Voltage and Current 2/2  "phase current 2"
  From13/1 -> transformer voltage and current 2/1  "transVotage2"
  Voltage Measurement6/1 -> Goto8/1
  Voltage Measurement9/1 -> Goto10/1
  Voltage Measurement10/1 -> Goto12/1
  From12/1 -> output voltages2/2  "bottom right voltage"
  From10/1 -> output voltages2/1  "upper right voltage"
  From8/1 -> output voltages1/3  "total left voltage"
  From4/1 -> output voltages1/1  "upper  left voltage"
  From9/1 -> output voltages1/2  "bottom left voltage"
  Constant2/1 -> "Pulse Generator (Thyristor, 6-Pulse)2"/1
  From7/1 -> Phase Voltage and Current 1/2  "phase current 1"
  "Pulse Generator (Thyristor, 6-Pulse)"/1 -> Goto/1
  Repeating Sequence/1 -> "Pulse Generator (Thyristor, 6-Pulse)"/2
  Voltage Measurement4/1 -> Goto4/1
  Voltage Measurement5/1 -> Display1/1, Goto6/1
  Voltage Measurement8/1 -> Goto9/1
  "Pulse Generator (Thyristor, 6-Pulse)2"/1 -> Goto2/1
  From6/1 -> Phase Voltage and Current 1/1  "phase voltage 1"
  From5/1 -> transformer voltage and current 1/1  "transVoltage1"
  Constant/1 -> "Pulse Generator (Thyristor, 6-Pulse)"/1
  From17/1 -> transformer voltage and current 1/2  "transCurrent1"
  From16/1 -> DC link current/1  "DC link current"
  Repeating Sequence2/1 -> "Pulse Generator (Thyristor, 6-Pulse)2"/2
  RMS12/1 -> Display17/1
  From18/1 -> transformer voltage and current 2/2  "transCurrent2"
  From14/1 -> Phase Voltage and Current 2/1  "phase voltage 2"
  Voltage Measurement/1 -> Goto3/1
  From1/1 -> Universal Bridge1/1
  From11/1 -> output voltages2/3  "total right voltage"
  From2/1 -> Universal Bridge2/1
  RMS13/1 -> Display/1
  From19/1 -> Universal Bridge4/1
  From20/1 -> Universal Bridge5/1
  From22/1 -> Universal Bridge7/1
  From24/1 -> Universal Bridge6/1
  From23/1 -> Universal Bridge/1
  Current Measurement1/1 -> Goto7/1
  Current Measurement3/1 -> Goto13/1
  Voltage Measurement3/1 -> Goto11/1
  "Pulse Generator (Thyristor, 6-Pulse)"/2 -> Goto16/1
  "Pulse Generator (Thyristor, 6-Pulse)2"/2 -> Goto18/1
  Current Measurement/1 -> Goto15/1
  Voltage Measurement1/1 -> Goto1/1
  Constant1/1 -> "Pulse Generator (Thyristor, 6-Pulse)1"/1
  Repeating Sequence1/1 -> "Pulse Generator (Thyristor, 6-Pulse)1"/2
  "Pulse Generator (Thyristor, 6-Pulse)1"/1 -> Universal Bridge8/1
  "Pulse Generator (Thyristor, 6-Pulse)1"/2 -> Universal Bridge9/1
  Constant3/1 -> Controlled Current Source/1
  Voltage Measurement7/1 -> Scope/1
  Voltage Measurement12/1 -> Scope2/1
  Voltage Measurement11/1 -> Scope1/1
  Voltage Measurement16/1 -> [phaseVoltage]
  DCcurrent1/1 -> RMS6/1, [DClinkCurrent]
  RMS6/1 -> Display2/1
  RMS2/1 -> Display7/1
  RMS4/1 -> Display9/1
  RMS5/1 -> Display8/1
  RMS3/1 -> Display4/1
  RMS9/1 -> Display3/1
  RMS7/1 -> Display6/1
  [ReceiverFiringAnglesY] -> Universal Bridge12/1
  [ReceiverFiringAnglesD] -> Universal Bridge13/1
  Voltage Measurement18/1 -> [VoltageSum1], RMS9/1
  Current Measurement2/1 -> [transCurrent1]
  [transCurrent2] -> transformer voltage2/2  "transCurrent2"
  [transCurrent1] -> transformer voltage1/2  "transCurrent1"
  Voltage Measurement13/1 -> [transVoltage1]
  [DClinkCurrent] -> DC link current1/1  "DC link current"
  [phaseCurrent2] -> Phase Voltage and Current 4/2  "phase current 2"
  [phaseVoltage2] -> Phase Voltage and Current 4/1  "phase voltage 2"
  Current Measurement6/1 -> [phaseCurrent2]
  Voltage Measurement19/1 -> [Voltage4], RMS2/1
  Voltage Measurement21/1 -> [transVoltage2]
  [transVoltage2] -> transformer voltage2/1  "transVotage2"
  Voltage Measurement22/1 -> [Voltage3], RMS5/1
  Voltage Measurement15/1 -> [VoltageSum2], RMS4/1
  [Voltage3] -> output voltages4/1  "upper right voltage"
  [Voltage4] -> output voltages4/2  "bottom right voltage"
  [VoltageSum2] -> output voltages4/3  "total right voltage"
  [VoltageSum1] -> output voltages3/3  "total left voltage"
  Voltage Measurement17/1 -> [Voltage1], RMS7/1
  [Voltage2] -> output voltages3/2  "bottom left voltage"
  [transVoltage1] -> transformer voltage1/1  "transVoltage1"
  [Voltage1] -> output voltages3/1  "upper  left voltage"
  Voltage Measurement14/1 -> [Voltage2], RMS3/1
  [phaseVoltage] -> Phase Voltage and Current 3/1  "phase voltage 1"
  [phaseCurrent] -> Phase Voltage and Current 3/2  "phase current 1"
  Constant5/1 -> "Pulse Generator (Thyristor, 6-Pulse)4"/1
  Repeating Sequence4/1 -> "Pulse Generator (Thyristor, 6-Pulse)4"/2
  "Pulse Generator (Thyristor, 6-Pulse)4"/1 -> [ReceiverFiringAnglesY]
  [SenderFiringAnglesD] -> Universal Bridge11/1
  "Pulse Generator (Thyristor, 6-Pulse)3"/1 -> [SenderFiringAnglesY]
  [SenderFiringAnglesY] -> Universal Bridge10/1
  Repeating Sequence3/1 -> "Pulse Generator (Thyristor, 6-Pulse)3"/2
  Constant4/1 -> "Pulse Generator (Thyristor, 6-Pulse)3"/1
  "Pulse Generator (Thyristor, 6-Pulse)3"/2 -> [SenderFiringAnglesD]
  "Pulse Generator (Thyristor, 6-Pulse)4"/2 -> [ReceiverFiringAnglesD]
  [SenderFiringAnglesY] -> Universal Bridge15/1
  [SenderFiringAnglesD] -> Universal Bridge14/1
  [ReceiverFiringAnglesD] -> Universal Bridge16/1
  [ReceiverFiringAnglesY] -> Universal Bridge17/1
  Current Measurement5/1 -> [transCurrent2]
  Voltage Measurement20/1 -> [phaseVoltage2]
  Current Measurement7/1 -> [phaseCurrent]
  [deltaCurrent] -> star and delta voltages/2  "delta current"
  [starCurrent] -> star and delta voltages/1  "star current"
  Current Measurement4/1 -> [starCurrent]
  Current Measurement8/1 -> [deltaCurrent]
  connections:
  Universal Bridge2/RConn2 -- Voltage Measurement9/LConn2 -- Voltage Measurement10/LConn2 -- DCcurrent/RConn1
  Universal Bridge1/RConn2 -- Voltage Measurement1/LConn2 -- Voltage Measurement5/LConn2 -- Series RLC Branch5/LConn1
  Series RLC Branch4/RConn1 -- Voltage Measurement10/LConn1 -- Voltage Measurement6/LConn1 -- Universal Bridge3/RConn1
  Current Measurement10/LConn1 -- Universal Bridge2/LConn3
  Series RLC Branch2/RConn1 -- DCcurrent/LConn1
  Series RLC Branch5/RConn1 -- Series RLC Branch1/LConn1
  Series RLC Branch4/LConn1 -- Series RLC Branch1/RConn1
  Series RLC Branch6/RConn1 -- Series RLC Branch/LConn1
  Series RLC Branch2/LConn1 -- Series RLC Branch/RConn1
  Series RLC Branch6/LConn1 -- Voltage Measurement5/LConn1 -- Voltage Measurement4/LConn1 -- Universal Bridge/RConn1
  Universal Bridge2/RConn1 -- Universal Bridge4/RConn2
  Universal Bridge4/RConn1 -- Voltage Measurement9/LConn1 -- Voltage Measurement6/LConn2 -- Universal Bridge5/RConn2 -- Ground1/LConn1
  Universal Bridge5/RConn1 -- Universal Bridge3/RConn2
  Three-Phase Programmable Voltage Source3/RConn2 -- Three-Phase Transformer (Three Windings)3/LConn2 -- Voltage Measurement3/LConn2
  Three-Phase Programmable Voltage Source3/RConn3 -- Three-Phase Transformer (Three Windings)3/LConn3
  Three-Phase Transformer (Three Windings)3/RConn1 -- Universal Bridge5/LConn1 -- Voltage Measurement8/LConn1 -- Universal Bridge2/LConn1
  Universal Bridge2/LConn2 -- Voltage Measurement8/LConn2 -- Three-Phase Transformer (Three Windings)3/RConn2 -- Universal Bridge5/LConn2
  Universal Bridge5/LConn3 -- Current Measurement10/RConn1 -- Three-Phase Transformer (Three Windings)3/RConn3
  Universal Bridge4/LConn1 -- Three-Phase Transformer (Three Windings)3/RConn4 -- Universal Bridge3/LConn1
  Universal Bridge3/LConn2 -- Universal Bridge4/LConn2 -- Three-Phase Transformer (Three Windings)3/RConn5
  Universal Bridge3/LConn3 -- Universal Bridge4/LConn3 -- Three-Phase Transformer (Three Windings)3/RConn6
  Three-Phase Programmable Voltage Source10/RConn2 -- Three-Phase Transformer (Three Windings)2/LConn2 -- Voltage Measurement2/LConn2
  Three-Phase Transformer (Three Windings)2/LConn3 -- Three-Phase Programmable Voltage Source10/RConn3
  Universal Bridge6/RConn2 -- Voltage Measurement4/LConn2 -- Voltage Measurement1/LConn1 -- Universal Bridge7/RConn1 -- Ground3/LConn1
  Universal Bridge/RConn2 -- Universal Bridge6/RConn1
  Universal Bridge7/RConn2 -- Universal Bridge1/RConn1
  Universal Bridge7/LConn1 -- Three-Phase Transformer (Three Windings)2/RConn1 -- Current Measurement/LConn1 -- Voltage Measurement/LConn1
  Three-Phase Transformer (Three Windings)2/RConn2 -- Universal Bridge7/LConn2 -- Universal Bridge/LConn2 -- Voltage Measurement/LConn2
  Universal Bridge7/LConn3 -- Three-Phase Transformer (Three Windings)2/RConn3 -- Universal Bridge/LConn3
  Universal Bridge6/LConn1 -- Three-Phase Transformer (Three Windings)2/RConn4 -- Universal Bridge1/LConn1
  Universal Bridge6/LConn2 -- Three-Phase Transformer (Three Windings)2/RConn5 -- Universal Bridge1/LConn2
  Universal Bridge1/LConn3 -- Three-Phase Transformer (Three Windings)2/RConn6 -- Universal Bridge6/LConn3
  Three-Phase Transformer (Three Windings)2/LConn1 -- Current Measurement1/RConn1
  Current Measurement1/LConn1 -- Voltage Measurement2/LConn1 -- Three-Phase Programmable Voltage Source10/RConn1
  Current Measurement3/LConn1 -- Three-Phase Transformer (Three Windings)3/LConn1
  Current Measurement3/RConn1 -- Three-Phase Programmable Voltage Source3/RConn1 -- Voltage Measurement3/LConn1
  Current Measurement/RConn1 -- Universal Bridge/LConn1
  Three-Phase Transformer (Three Windings)1/RConn1 -- Voltage Measurement7/LConn1 -- Universal Bridge8/LConn1
  Three-Phase Transformer (Three Windings)1/RConn2 -- Voltage Measurement7/LConn2 -- Universal Bridge8/LConn2
  Three-Phase Transformer (Three Windings)1/RConn3 -- Universal Bridge8/LConn3
  Universal Bridge8/RConn2 -- Universal Bridge9/RConn1
  Ground/LConn1 -- Voltage Measurement12/LConn2 -- Controlled Current Source/RConn1 -- Universal Bridge9/RConn2
  Controlled Current Source/LConn1 -- Voltage Measurement12/LConn1 -- Universal Bridge8/RConn1
  Three-Phase Transformer (Three Windings)1/RConn4 -- Voltage Measurement11/LConn1 -- Universal Bridge9/LConn1
  Three-Phase Transformer (Three Windings)1/RConn5 -- Voltage Measurement11/LConn2 -- Universal Bridge9/LConn2
  Three-Phase Transformer (Three Windings)1/RConn6 -- Universal Bridge9/LConn3
  Three-Phase Programmable Voltage Source1/RConn1 -- Three-Phase Transformer (Three Windings)1/LConn1
  Three-Phase Programmable Voltage Source1/RConn2 -- Three-Phase Transformer (Three Windings)1/LConn2
  Three-Phase Programmable Voltage Source1/RConn3 -- Three-Phase Transformer (Three Windings)1/LConn3
  Series RLC Branch11/LConn1 -- Series RLC Branch10/RConn1
  Series RLC Branch10/LConn1 -- Series RLC Branch9/RConn1
  Universal Bridge10/LConn2 -- Three-Phase Transformer (Two Windings)23/RConn2
  Voltage Measurement13/LConn1 -- Universal Bridge10/LConn1 -- Current Measurement2/RConn1
  Universal Bridge11/RConn2 -- Series RLC Branch12/LConn1 -- Voltage Measurement14/LConn2 -- Voltage Measurement18/LConn2
  Voltage Measurement17/LConn1 -- Universal Bridge10/RConn1 -- Voltage Measurement18/LConn1 -- Series RLC Branch14/LConn1
  Universal Bridge10/RConn2 -- Universal Bridge14/RConn1
  Current Measurement6/RConn1 -- Three-Phase Transformer (Two Windings)8/RConn3 -- Three-Phase Transformer (Two Windings)1/RConn3
  Universal Bridge12/RConn2 -- Voltage Measurement22/LConn2 -- Voltage Measurement15/LConn2 -- DCcurrent1/RConn1
  Universal Bridge17/RConn1 -- Universal Bridge13/RConn2
  Three-Phase Programmable Voltage Source2/RConn2 -- Three-Phase Transformer (Two Windings)23/LConn2 -- Three-Phase Transformer (Two Windings)4/LConn2 -- Three-Phase Transformer (Two Windings)17/LConn2 -- Three-Phase Transformer (Two Windings)7/LConn2
  Voltage Measurement16/LConn1 -- Three-Phase Programmable Voltage Source2/RConn1 -- Current Measurement7/LConn1
  Three-Phase Programmable Voltage Source2/RConn3 -- Three-Phase Transformer (Two Windings)23/LConn3 -- Three-Phase Transformer (Two Windings)4/LConn3 -- Three-Phase Transformer (Two Windings)17/LConn3 -- Three-Phase Transformer (Two Windings)7/LConn3
  Three-Phase Transformer (Two Windings)6/RConn2 -- Three-Phase Programmable Voltage Source4/RConn2 -- Three-Phase Transformer (Two Windings)2/RConn2 -- Three-Phase Transformer (Two Windings)8/RConn2 -- Three-Phase Transformer (Two Windings)1/RConn2
  Series RLC Branch13/RConn1 -- Voltage Measurement15/LConn1 -- Voltage Measurement19/LConn1 -- Universal Bridge13/RConn1
  Voltage Measurement21/LConn1 -- Three-Phase Transformer (Two Windings)1/LConn1 -- Universal Bridge12/LConn1
  Three-Phase Transformer (Two Windings)1/LConn2 -- Universal Bridge12/LConn2
  Current Measurement6/LConn1 -- Three-Phase Transformer (Two Windings)2/RConn3 -- Three-Phase Transformer (Two Windings)6/RConn3 -- Three-Phase Programmable Voltage Source4/RConn3
  Three-Phase Transformer (Two Windings)8/LConn2 -- Universal Bridge13/LConn2
  Three-Phase Transformer (Two Windings)8/LConn3 -- Universal Bridge13/LConn3
  Three-Phase Transformer (Two Windings)8/LConn1 -- Universal Bridge13/LConn1
  Current Measurement2/LConn1 -- Three-Phase Transformer (Two Windings)23/RConn1
  Series RLC Branch12/RConn1 -- Series RLC Branch7/LConn1
  Series RLC Branch14/RConn1 -- Series RLC Branch3/LConn1
  Series RLC Branch13/LConn1 -- Series RLC Branch7/RConn1
  Series RLC Branch8/LConn1 -- Series RLC Branch3/RConn1
  Three-Phase Programmable Voltage Source4/RConn1 -- Three-Phase Transformer (Two Windings)6/RConn1 -- Three-Phase Transformer (Two Windings)2/RConn1 -- Three-Phase Transformer (Two Windings)8/RConn1 -- Three-Phase Transformer (Two Windings)1/RConn1 -- Voltage Measurement20/LConn1
  Series RLC Branch8/RConn1 -- DCcurrent1/LConn1
  Universal Bridge10/LConn3 -- Three-Phase Transformer (Two Windings)23/RConn3
  Three-Phase Transformer (Two Windings)17/RConn1 -- Universal Bridge11/LConn1
  Three-Phase Transformer (Two Windings)17/RConn2 -- Universal Bridge11/LConn2
  Three-Phase Transformer (Two Windings)17/RConn3 -- Universal Bridge11/LConn3
  Universal Bridge15/RConn2 -- Universal Bridge11/RConn1
  Universal Bridge14/RConn2 -- Voltage Measurement14/LConn1 -- Universal Bridge15/RConn1 -- Ground4/LConn1 -- Voltage Measurement17/LConn2
  Three-Phase Transformer (Two Windings)4/RConn3 -- Universal Bridge14/LConn3
  Three-Phase Transformer (Two Windings)4/RConn2 -- Universal Bridge14/LConn2
  Three-Phase Transformer (Two Windings)4/RConn1 -- Universal Bridge14/LConn1
  Three-Phase Transformer (Two Windings)7/RConn1 -- Universal Bridge15/LConn1
  Three-Phase Transformer (Two Windings)7/RConn2 -- Universal Bridge15/LConn2
  Three-Phase Transformer (Two Windings)7/RConn3 -- Universal Bridge15/LConn3
  Three-Phase Transformer (Two Windings)2/LConn3 -- Universal Bridge16/LConn3
  Three-Phase Transformer (Two Windings)2/LConn2 -- Universal Bridge16/LConn2
  Three-Phase Transformer (Two Windings)2/LConn1 -- Universal Bridge16/LConn1
  Three-Phase Transformer (Two Windings)6/LConn3 -- Universal Bridge17/LConn3
  Three-Phase Transformer (Two Windings)6/LConn2 -- Universal Bridge17/LConn2
  Three-Phase Transformer (Two Windings)6/LConn1 -- Universal Bridge17/LConn1
  Universal Bridge12/RConn1 -- Universal Bridge16/RConn2
  Ground2/LConn1 -- Voltage Measurement19/LConn2 -- Universal Bridge17/RConn2 -- Universal Bridge16/RConn1 -- Voltage Measurement22/LConn1
  Current Measurement5/LConn1 -- Universal Bridge12/LConn3
  Three-Phase Transformer (Two Windings)1/LConn3 -- Current Measurement5/RConn1
  Voltage Measurement16/LConn2 -- Three-Phase Programmable Voltage Source2/LConn1
  Voltage Measurement20/LConn2 -- Three-Phase Programmable Voltage Source4/LConn1
  Three-Phase Transformer (Two Windings)1/LConn4 -- Voltage Measurement21/LConn2
  Voltage Measurement13/LConn2 -- Three-Phase Transformer (Two Windings)23/RConn4
  Three-Phase Transformer (Two Windings)17/LConn1 -- Three-Phase Transformer (Two Windings)7/LConn1 -- Current Measurement8/LConn1 -- Current Measurement4/LConn1 -- Current Measurement7/RConn1
  Current Measurement4/RConn1 -- Three-Phase Transformer (Two Windings)23/LConn1
  Three-Phase Transformer (Two Windings)4/LConn1 -- Current Measurement8/RConn1
